simulink model "SebessegOszekapcsolasaSzemletetes"  (R2014a)
settings: Solver=ode45  StartTime=0.0  StopTime=10.0  RelTol=1e-3
settings Model: Creator=laca  LastModifiedBy=laca

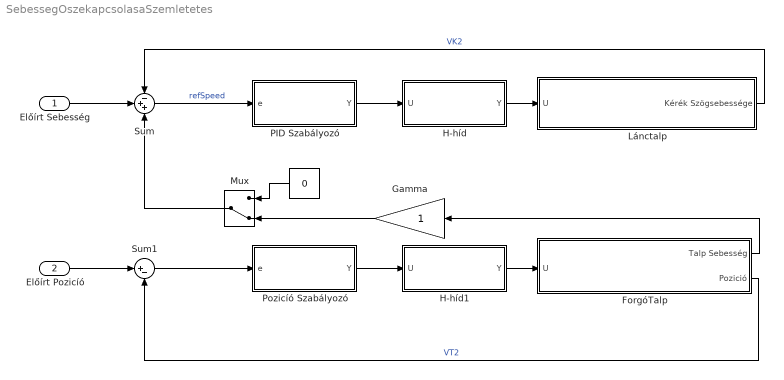
== system SebessegOszekapcsolasaSzemletetes ==
  Előírt Sebesség : Inport
  Előírt Pozicíó : Inport  Port=2
  " " : Constant  Value=0
  ForgóTalp : Subsystem
  Gamma : Gain
  H-híd : Subsystem
  H-híd1 : Subsystem
  Lánctalp : Subsystem
  Mux : ManualSwitch  CurrentSetting=0
  PID Szabályozó : Subsystem
  Pozicíó Szabályozó : Subsystem
  Sum : Sum  Inputs=-++
  Sum1 : Sum  Inputs=|+-
  wires:
  PID Szabályozó/1(Y) -> H-híd/1(U)
  Sum/1 -> PID Szabályozó/1(e)  "refSpeed"
  Lánctalp/1(Kérék Szögsebessége) -> Sum/1  "VK2"
  Pozicíó Szabályozó/1(Y) -> H-híd1/1(U)
  H-híd1/1(Y) -> ForgóTalp/1(U)
  Sum1/1 -> Pozicíó Szabályozó/1(e)
  ForgóTalp/1(Talp Sebesség) -> Gamma/1
  ForgóTalp/2(Pozició) -> Sum1/2  "VT2"
  H-híd/1(Y) -> Lánctalp/1(U)
  Mux/1 -> Sum/3
  " "/1 -> Mux/1
  Gamma/1 -> Mux/2
  Előírt Sebesség/1 -> Sum/2
  Előírt Pozicíó/1 -> Sum1/1

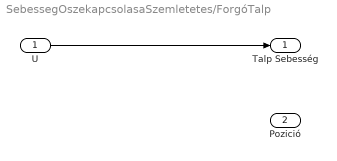
== system SebessegOszekapcsolasaSzemletetes/ForgóTalp ==
  U : Inport
  Talp Sebesség : Outport
  Pozició : Outport  Port=2
  wires:
  U/1 -> Talp Sebesség/1

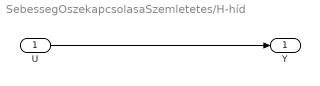
== system SebessegOszekapcsolasaSzemletetes/H-híd ==
  U : Inport
  Y : Outport
  wires:
  U/1 -> Y/1

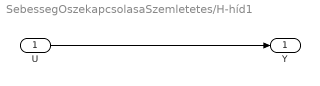
== system SebessegOszekapcsolasaSzemletetes/H-híd1 ==
  U : Inport
  Y : Outport
  wires:
  U/1 -> Y/1

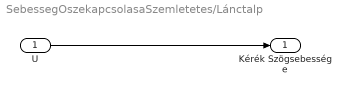
== system SebessegOszekapcsolasaSzemletetes/Lánctalp ==
  U : Inport
  Kérék Szögsebessége : Outport
  wires:
  U/1 -> Kérék Szögsebessége/1

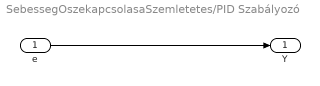
== system SebessegOszekapcsolasaSzemletetes/PID Szabályozó ==
  e : Inport
  Y : Outport
  wires:
  e/1 -> Y/1

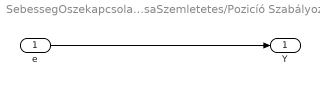
== system SebessegOszekapcsolasaSzemletetes/Pozicíó Szabályozó ==
  e : Inport
  Y : Outport
  wires:
  e/1 -> Y/1
